simulink model "task1"  (R2022a)
settings: Solver=FixedStepAuto  StartTime=0.0  StopTime=1  FixedStep=10e-4  RelTol=1e-3
values from neighbouring files (symbols this model uses):
  K = 99.4473654351    [K.mat]    (also in K1.mat = 13.0862573698)
  K1 = 13.0862573698    [K1.mat]
  T1 = 0.02    [K.mat]    (also in K1.mat)
  T2 = 0.002    [K.mat]    (also in K1.mat)
settings Model: Creator=mikol  LastModifiedBy=mikol

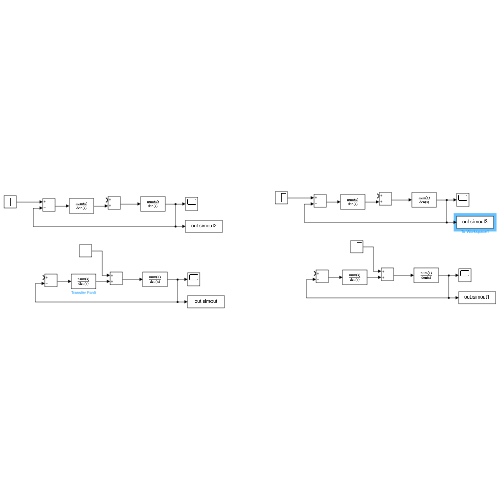
[thumbnail: Simulink's stored preview of the top-level diagram]
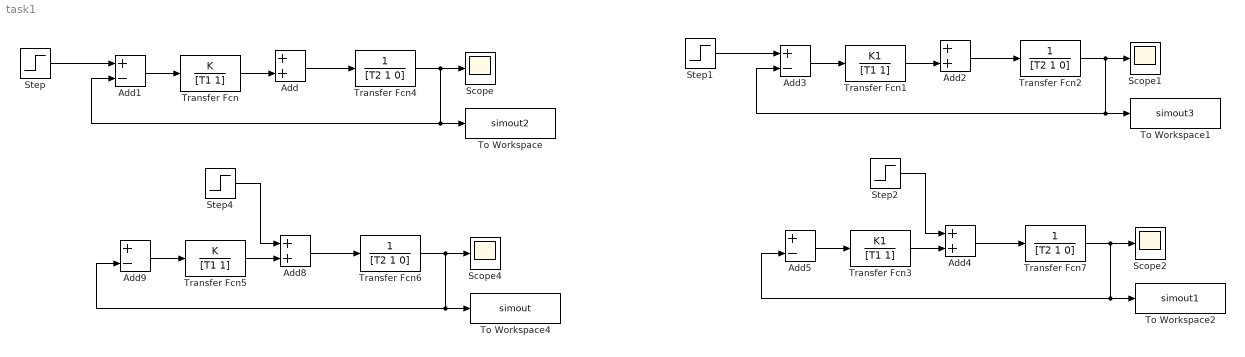
== system task1 ==
  Add{,2,4,8} (4 alike) : Sum
  Add{1,3,5,9} (4 alike) : Sum  Inputs=+-
  Scope{,1..2,4} (4 alike) : Scope
  Step{,1..2,4} (4 alike) : Step  Time=0  SampleTime=0
  To Workspace : ToWorkspace  VariableName=simout2  SampleTime=-1
      settings: Save2DSignal=2-D array (concatenate along first dimension)
  To Workspace1 : ToWorkspace  VariableName=simout3  SampleTime=-1
      settings: Save2DSignal=2-D array (concatenate along first dimension)
  To Workspace2 : ToWorkspace  VariableName=simout1  SampleTime=-1
      settings: Save2DSignal=2-D array (concatenate along first dimension)
  To Workspace4 : ToWorkspace  VariableName=simout  SampleTime=-1
      settings: Save2DSignal=2-D array (concatenate along first dimension)
  Transfer Fcn : TransferFcn  Numerator=K  Denominator=[T1 1]
  Transfer Fcn1 : TransferFcn  Numerator=K1  Denominator=[T1 1]
  Transfer Fcn{2,4,6..7} (4 alike) : TransferFcn  Denominator=[T2 1 0]
  Transfer Fcn3 : TransferFcn  Numerator=K1  Denominator=[T1 1]
  Transfer Fcn5 : TransferFcn  Numerator=K  Denominator=[T1 1]
  wires:
  Transfer Fcn/1 -> Add/2
  Add1/1 -> Transfer Fcn/1
  Add/1 -> Transfer Fcn4/1
  Transfer Fcn4/1 -> Add1/2, To Workspace/1, Scope/1
  Add8/1 -> Transfer Fcn6/1
  Transfer Fcn6/1 -> Add9/2, To Workspace4/1, Scope4/1
  Step4/1 -> Add8/1
  Add9/1 -> Transfer Fcn5/1
  Transfer Fcn5/1 -> Add8/2
  Step/1 -> Add1/1
  Step1/1 -> Add3/1
  Step2/1 -> Add4/1
  Transfer Fcn3/1 -> Add4/2
  Transfer Fcn7/1 -> Add5/2, To Workspace2/1, Scope2/1
  Add2/1 -> Transfer Fcn2/1
  Add5/1 -> Transfer Fcn3/1
  Transfer Fcn2/1 -> Add3/2, To Workspace1/1, Scope1/1
  Add4/1 -> Transfer Fcn7/1
  Add3/1 -> Transfer Fcn1/1
  Transfer Fcn1/1 -> Add2/2
